simulink model "compassGaitSim_impacts3"  (R2013a)
settings: Solver=ode45  StartTime=0.0  StopTime=5  FixedStep=0.01  MaxStep=0.02  MinStep=1e-16  RelTol=1e-3
values from neighbouring files (symbols this model uses):
  g = 9.81    [runSim.m]
  I1 = Is(1)    [PartialSolZeroDyn.m]    (also in impactDynamics_broken.m; runSim.m = 1)
  I2 = Is(2)    [PartialSolZeroDyn.m]    (also in impactDynamics_broken.m; runSim.m = 0.6)
  l1 = ls(1)    [PartialSolZeroDyn.m]    (also in impactDynamics_broken.m; runSim.m = 0.5)
  l2 = ls(2)    [PartialSolZeroDyn.m]    (also in impactDynamics_broken.m; runSim.m = 0.5)
  m1 = ms(1)    [PartialSolZeroDyn.m]    (also in impactDynamics_broken.m; runSim.m = 1.2)
  m2 = ms(2)    [PartialSolZeroDyn.m]    (also in impactDynamics_broken.m; runSim.m = 1.2)
  points = get(handles.uitable1, 'Data')'    [BezGui.m]    (also in BezGuiAttempt.m = [P0'; P1'; P2'; P3']; runSim.m = BezGuiAttempt')
undefined symbols (not defined in the file or in its folder): t1_0, t1d_0, t2_0, t2d_0
libraries: simulink x2, dspsigops x1
settings Model: CovHTMLOptions=-sRT=1 -aTS=1 -bRG=1 -bTC=1 -hTR=0 -nFC=0 -scm=1 -bcm=1 -xEv=0  Creator=yak  LastModifiedBy=yak
settings SolverCC: MaxConsecutiveMinStep=10
settings DataIOCC: LimitDataPoints=off  OutputOption=SpecifiedOutputTimes  OutputTimes=0:0.01:(timeleft-0.01)
settings DebuggingCC: DiscreteInheritContinuousMsg=none  MultiTaskDSMMsg=warning  MultiTaskCondExecSysMsg=none  FcnCallInpInsideContextMsg=EnableAllAsWarning  StrictBusMsg=None
settings RTWCC: IncludeERTFirstTime=on

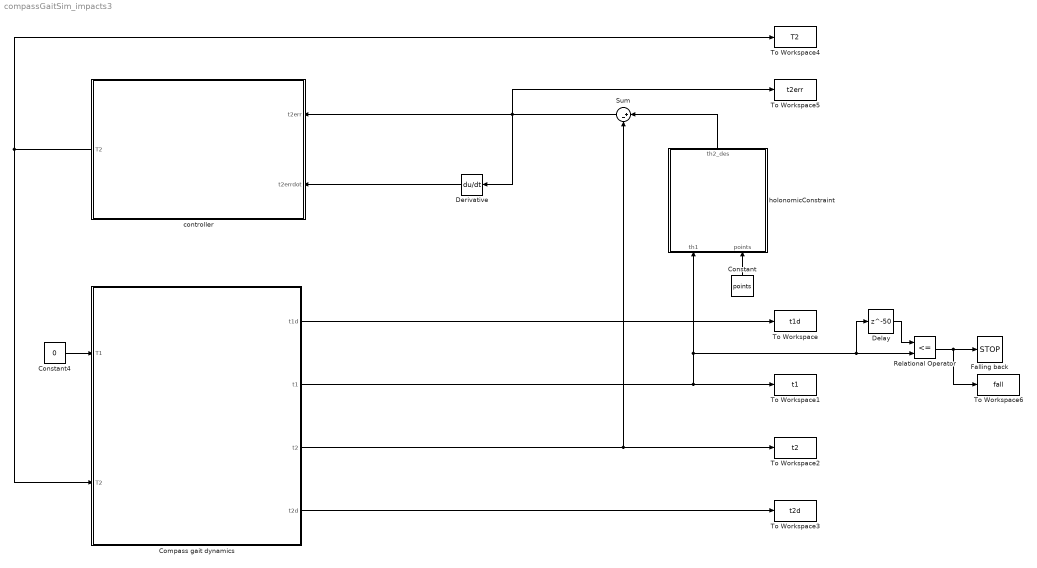
== system compassGaitSim_impacts3 ==
  Compass gait dynamics : Subsystem
  Constant : Constant  Value=points
  Constant4 : Constant  Value=0
  Delay : Delay  DelayLength=50  InitialCondition=100  SampleTime=0.01
  Derivative : Derivative
  Falling back : Stop
  Relational Operator : RelationalOperator  Operator=<=  OutDataTypeStr=boolean  ZeroCross=off
  Sum : Sum  Inputs=|+-
  To Workspace : ToWorkspace  VariableName=t1d  SampleTime=-1
  To Workspace1 : ToWorkspace  VariableName=t1  SampleTime=-1
  To Workspace2 : ToWorkspace  VariableName=t2  SampleTime=-1
  To Workspace3 : ToWorkspace  VariableName=t2d  SampleTime=-1
  To Workspace4 : ToWorkspace  VariableName=T2  SampleTime=-1
  To Workspace5 : ToWorkspace  VariableName=t2err  SampleTime=-1
  To Workspace6 : ToWorkspace  VariableName=fall  SampleTime=-1
      settings: MaxDataPoints=1
  controller : MATLAB Function  TreatAsAtomicUnit=on
  holonomicConstraint : MATLAB Function  TreatAsAtomicUnit=on
  wires:
  controller/1(T2) -> Compass gait dynamics/2(T2), To Workspace4/1
  Compass gait dynamics/1(t1d) -> To Workspace/1
  Compass gait dynamics/2(t1) -> To Workspace1/1, Delay/1, Relational Operator/2, holonomicConstraint/1(th1)
  Compass gait dynamics/3(t2) -> Sum/2, To Workspace2/1
  Compass gait dynamics/4(t2d) -> To Workspace3/1
  Constant4/1 -> Compass gait dynamics/1(T1)
  holonomicConstraint/1(th2_des) -> Sum/1
  Sum/1 -> To Workspace5/1, Derivative/1, controller/1(t2err)
  Derivative/1 -> controller/2(t2errdot)
  Constant/1 -> holonomicConstraint/2(points)
  Delay/1 -> Relational Operator/1
  Relational Operator/1 -> To Workspace6/1, Falling back/1

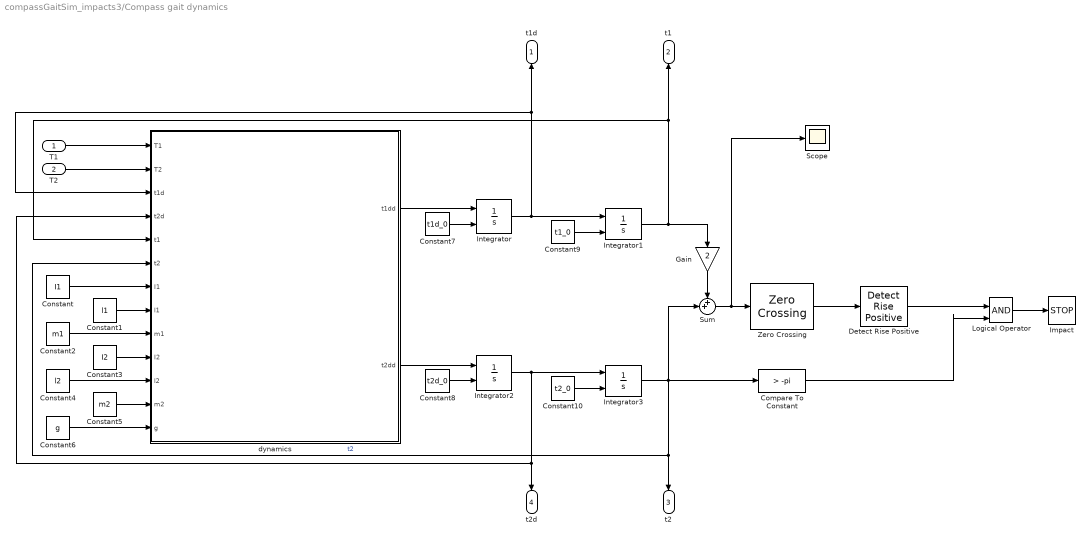
== system compassGaitSim_impacts3/Compass gait dynamics ==
  T1 : Inport
  T2 : Inport  Port=2
  Compare To Constant : simulink/Logic and Bit Operations/Compare To Constant  relop=>  const=-pi  OutDataTypeStr=boolean  ZeroCross=off
  Constant : Constant  Value=I1
  Constant1 : Constant  Value=l1
  Constant10 : Constant  Value=t2_0
  Constant2 : Constant  Value=m1
  Constant3 : Constant  Value=I2
  Constant4 : Constant  Value=l2
  Constant5 : Constant  Value=m2
  Constant6 : Constant  Value=g
  Constant7 : Constant  Value=t1d_0
  Constant8 : Constant  Value=t2d_0
  Constant9 : Constant  Value=t1_0
  Detect Rise Positive : simulink/Logic and Bit Operations/Detect Rise Positive  vinit=0  InputProcessing=Inherited  OutDataTypeStr=boolean
  Gain : Gain  Gain=2
  Impact : Stop
  Integrator{,1..3} (4 alike) : Integrator  InitialConditionSource=external
  Logical Operator : Logic  IconShape=distinctive  AllPortsSameDT=off  OutDataTypeStr=boolean
  Scope : Scope
  Sum : Sum  Inputs=++|
  Zero Crossing : dspsigops/Zero Crossing  InputProcessing=Columns as channels (frame based)
  dynamics : MATLAB Function  TreatAsAtomicUnit=on
  t1d : Outport
  t1 : Outport  Port=2
  t2 : Outport  Port=3
  t2d : Outport  Port=4
  wires:
  T1/1 -> dynamics/1(T1)
  T2/1 -> dynamics/2(T2)
  dynamics/1(t1dd) -> Integrator/1
  Integrator/1 -> t1d/1, dynamics/3(t1d), Integrator1/1
  Integrator2/1 -> t2d/1, dynamics/4(t2d), Integrator3/1
  Integrator3/1 -> Compare To Constant/1, t2/1, dynamics/6(t2), Sum/2  "t2"
  Integrator1/1 -> dynamics/5(t1), t1/1, Gain/1
  Constant2/1 -> dynamics/9(m1)
  Constant/1 -> dynamics/7(I1)
  Constant1/1 -> dynamics/8(l1)
  Constant3/1 -> dynamics/10(I2)
  Constant4/1 -> dynamics/11(l2)
  Constant5/1 -> dynamics/12(m2)
  Constant6/1 -> dynamics/13(g)
  Constant7/1 -> Integrator/2
  Constant9/1 -> Integrator1/2
  dynamics/2(t2dd) -> Integrator2/1
  Logical Operator/1 -> Impact/1
  Constant8/1 -> Integrator2/2
  Constant10/1 -> Integrator3/2
  Sum/1 -> Scope/1, Zero Crossing/1
  Gain/1 -> Sum/1
  Zero Crossing/1 -> Detect Rise Positive/1
  Compare To Constant/1 -> Logical Operator/2
  Detect Rise Positive/1 -> Logical Operator/1

== matlab function compassGaitSim_impacts3/controller ==
  data: t2err input; t2errdot input; T2 output
function T2 = controller(t2err, t2errdot)
%#codegen

% Simple PD controller:
K_p = 1000;
K_d = 100;

t2err = mod(t2err, 2*pi);   % Ensure error is within 1 rotation

% Ensure error is in the range [-pi pi]
if t2err > pi
    t2err = -(2*pi - t2err);
elseif t2err < -pi
    t2err = 2*pi - t2err;
end

T2 = K_p*t2err + K_d*t2errdot;
% TODO: Add zero dynamics to controller


end

== matlab function compassGaitSim_impacts3/Compass gait dynamics/dynamics ==
  data: T1 input; t1dd output; T2 input; t1d input; t2d input; t1 input; t2 input; t2dd output; I1 input; l1 input; m1 input; I2 input; l2 input; m2 input; g input
function [t1dd, t2dd] = compassGaitDynamics(T1, T2, t1d, t2d, t1, t2, ...
    I1, l1, m1, I2, l2, m2, g)
%#codegen

c1 = cos(t1);
c2 = cos(t2);
s2 = sin(t2);
c12 = cos(t1 + t2);


% Equations in terms of T1 and T2 are derived, then the solution in terms
% of the angle accelerations have been pre-solved. The output is below.
t1dd = (4*I2*T1 - 4*I2*T2 + T1*l2^2*m2 - T2*l2^2*m2 - ...
    c1*g*l1*l2^2*m2^2 - 2*I2*c1*g*l1*m1 - 4*I2*c1*g*l1*m2 - ...
    2*T2*c2*l1*l2*m2 + (l1*l2^3*m2^2*s2*t1d^2)/2 + ...
    (l1*l2^3*m2^2*s2*t2d^2)/2 + 2*I2*l1*l2*m2*s2*t1d^2 + ...
    2*I2*l1*l2*m2*s2*t2d^2 - (c1*g*l1*l2^2*m1*m2)/2 + ...
    c2*l1^2*l2^2*m2^2*s2*t1d^2 + c2*c12*g*l1*l2^2*m2^2 + ...
    l1*l2^3*m2^2*s2*t1d*t2d + 4*I2*l1*l2*m2*s2*t1d*t2d)/ ...
    (- c2^2*l1^2*l2^2*m2^2 + l1^2*l2^2*m2^2 + ...
    4*I2*l1^2*m2 + I1*l2^2*m2 + 4*I1*I2);

t2dd = -(4*I2*T1 - 4*I1*T2 - 4*I2*T2 + T1*l2^2*m2 - 4*T2*l1^2*m2 - ...
    T2*l2^2*m2 - c1*g*l1*l2^2*m2^2 + 2*c12*g*l1^2*l2*m2^2 - ...
    2*I2*c1*g*l1*m1 - 4*I2*c1*g*l1*m2 + 2*I1*c12*g*l2*m2 + ...
    2*T1*c2*l1*l2*m2 - 4*T2*c2*l1*l2*m2 + (l1*l2^3*m2^2*s2*t1d^2)/2 + ...
    2*l1^3*l2*m2^2*s2*t1d^2 + (l1*l2^3*m2^2*s2*t2d^2)/2 + ...
    2*I1*l1*l2*m2*s2*t1d^2 + 2*I2*l1*l2*m2*s2*t1d^2 + ...
    2*I2*l1*l2*m2*s2*t2d^2 - (c1*g*l1*l2^2*m1*m2)/2 + ...
    2*c2*l1^2*l2^2*m2^2*s2*t1d^2 + c2*l1^2*l2^2*m2^2*s2*t2d^2 - ...
    2*c1*c2*g*l1^2*l2*m2^2 + c2*c12*g*l1*l2^2*m2^2 + ...
    l1*l2^3*m2^2*s2*t1d*t2d + 4*I2*l1*l2*m2*s2*t1d*t2d + ...
    2*c2*l1^2*l2^2*m2^2*s2*t1d*t2d - c1*c2*g*l1^2*l2*m1*m2)/(- ...
    c2^2*l1^2*l2^2*m2^2 + l1^2*l2^2*m2^2 + 4*I2*l1^2*m2 + I1*l2^2*m2 + ...
    4*I1*I2);

end

== matlab function compassGaitSim_impacts3/holonomicConstraint ==
  data: th1 input; points input; th2_des output
function th2_des = holonomicConstraint(th1, points)
%#codegen

t = (th1 - points(1,1)) / (points(end,1) - points(1,1));

if t > 1
    t = 1;
elseif t < 0
    t = 0;
end

th2_des = 0;
n = size(points, 1) - 1;
for i = 0 : n
    th2_des = th2_des + nchoosek(n,i) * (1-t)^(n-i) * t^i * points(i+1,2);
end

end
